simulink model "requriment_33"  (R2021a)
settings: Solver=FixedStepDiscrete  StartTime=0.0  StopTime=50  FixedStep=1  RelTol=1e-3
libraries: simulink x12
settings Model: DataDictionary=requriment_33.sldd  Creator=Rahul  LastModifiedBy=Rahul
settings ConfigComp: CovMetricSettings=dcmwe

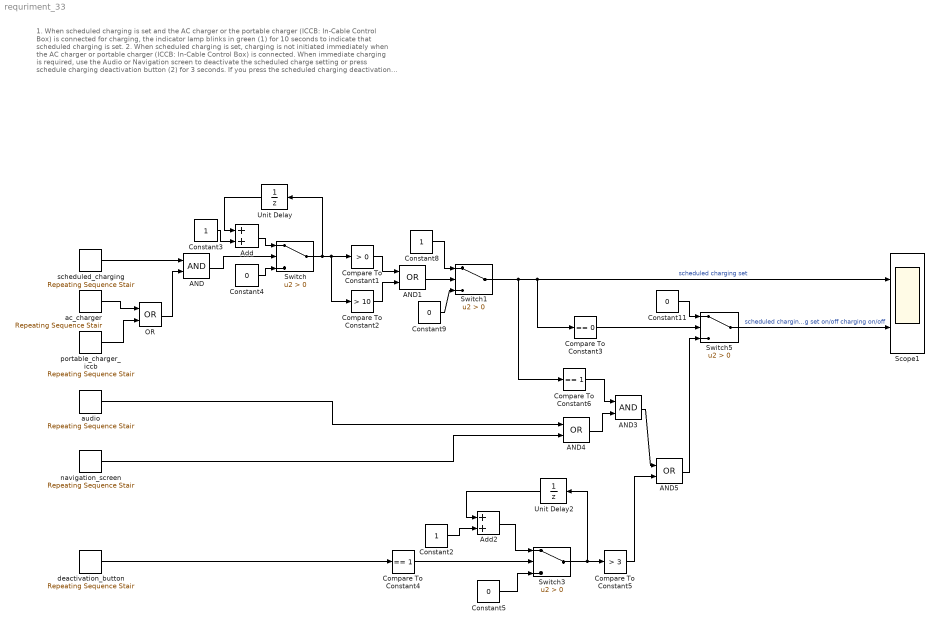
== system requriment_33 ==
  note: 1. When scheduled charging is set and the AC charger or the portable charger (ICCB: In-Cable Control Box) is connected for charging, the indicator lamp blinks in green (1) for 10 seconds to indicate
      | that scheduled charging is set.
      | 2. When scheduled charging is set, charging is not initiated immediately when the AC charger or portable charger (ICCB: In-Cable Control Box) is connected. When immediate charging is required,
      | use the Audio or Navigation screen to deactivate the scheduled charge setting
      | or press schedule charging deactivation button (2) for 3 seconds.
      | If you press the scheduled charging deactivation button (2) to immediately charge the battery,
      | charging must be initiated 3 minutes after the charging cable has been connected. When you press the scheduled charging deactivation button (2) for immediate charging, the schedul ed
      | charge setting
  AND : Logic  AllPortsSameDT=off  OutDataTypeStr=boolean
  AND1 : Logic  Operator=OR  AllPortsSameDT=off  OutDataTypeStr=boolean
  AND3 : Logic  AllPortsSameDT=off  OutDataTypeStr=boolean
  AND4 : Logic  Operator=OR  AllPortsSameDT=off  OutDataTypeStr=boolean
  AND5 : Logic  Operator=OR  AllPortsSameDT=off  OutDataTypeStr=boolean
  Add : Sum
  Add2 : Sum
  Compare To Constant1 : simulink/Logic and Bit Operations/Compare To Constant  relop=>  const=0  OutDataTypeStr=boolean
  Compare To Constant2 : simulink/Logic and Bit Operations/Compare To Constant  relop=>  const=10  OutDataTypeStr=boolean
  Compare To Constant3 : simulink/Logic and Bit Operations/Compare To Constant  relop===  const=0  OutDataTypeStr=boolean
  Compare To Constant4 : simulink/Logic and Bit Operations/Compare To Constant  relop===  const=1  OutDataTypeStr=boolean
  Compare To Constant5 : simulink/Logic and Bit Operations/Compare To Constant  relop=>  const=3  OutDataTypeStr=boolean
  Compare To Constant6 : simulink/Logic and Bit Operations/Compare To Constant  relop===  const=1  OutDataTypeStr=boolean
  Constant{4..5,9,11} (4 alike) : Constant  Value=0
  Constant2 : Constant
  Constant3 : Constant
  Constant8 : Constant
  OR : Logic  Operator=OR  AllPortsSameDT=off  OutDataTypeStr=boolean
  Scope1 : Scope  NumInputPorts=2
  Switch{,1,3,5} (4 alike) : Switch  Criteria=u2 > Threshold
  Unit Delay : UnitDelay  SampleTime=-1  HasFrameUpgradeWarning=on
  Unit Delay2 : UnitDelay  SampleTime=-1  HasFrameUpgradeWarning=on
  ac_charger : simulink/Sources/Repeating Sequence Stair  OutValues=[1 1 1 1 1 1 1 1 1 1 1 0 1 1 0 0 10 1 0 1 0 0 0 0]  tsamp=-1  OutMin=[]  OutMax=[]  OutDataTypeStr=double  OutputDataTypeScalingMode=double  OutDataType=fixdt(0,8)  ConRadixGroup=Best Precision: Vector-wise  OutScaling=2^-12
  audio : simulink/Sources/Repeating Sequence Stair  OutValues="[1 1 1 1 1 1 1 1 1 1 1 1 1 1 0 0 0  0 0 0  0 0 0 0]"  tsamp=-1  OutMin=[]  OutMax=[]  OutDataTypeStr=double  OutputDataTypeScalingMode=double  OutDataType=fixdt(0,8)  ConRadixGroup=Best Precision: Vector-wise  OutScaling=2^-12
  deactivation_button : simulink/Sources/Repeating Sequence Stair  OutValues="[1 1 1 1 1 1 1 1 1 1 1 1 1 1 0 0 0  0 0 0  0 0 0 0]"  tsamp=-1  OutMin=[]  OutMax=[]  OutDataTypeStr=double  OutputDataTypeScalingMode=double  OutDataType=fixdt(0,8)  ConRadixGroup=Best Precision: Vector-wise  OutScaling=2^-12
  navigation_screen : simulink/Sources/Repeating Sequence Stair  OutValues="[1 1 1 1 1 1 1 1 1 1 1 1 1 1 0 0 0  0 0 0  0 0 0 0]"  tsamp=-1  OutMin=[]  OutMax=[]  OutDataTypeStr=double  OutputDataTypeScalingMode=double  OutDataType=fixdt(0,8)  ConRadixGroup=Best Precision: Vector-wise  OutScaling=2^-12
  portable_charger_iccb : simulink/Sources/Repeating Sequence Stair  OutValues=[1 1 1 1 1 1 1 1 1 1 1 0 1 1 0 0 10 1 0 1 0 0 0 0]  tsamp=-1  OutMin=[]  OutMax=[]  OutDataTypeStr=double  OutputDataTypeScalingMode=double  OutDataType=fixdt(0,8)  ConRadixGroup=Best Precision: Vector-wise  OutScaling=2^-12
  scheduled_charging : simulink/Sources/Repeating Sequence Stair  OutValues=[1 1 1 1 1 1 1 1 1 1 1 1 1 1 0 0 10 1 0 1 0 0 0 0]  tsamp=-1  OutMin=[]  OutMax=[]  OutDataTypeStr=double  OutputDataTypeScalingMode=double  OutDataType=fixdt(0,8)  ConRadixGroup=Best Precision: Vector-wise  OutScaling=2^-12
  wires:
  Constant4/1 -> Switch/3
  ac_charger/1 -> OR/1
  portable_charger_iccb/1 -> OR/2
  AND/1 -> Switch/2
  scheduled_charging/1 -> AND/1
  Add/1 -> Switch/1
  OR/1 -> AND/2
  Constant3/1 -> Add/2
  Unit Delay/1 -> Add/1
  AND1/1 -> Switch1/2
  Constant9/1 -> Switch1/3
  Constant8/1 -> Switch1/1
  Compare To Constant1/1 -> AND1/1
  Compare To Constant2/1 -> AND1/2
  Switch/1 -> Compare To Constant2/1, Compare To Constant1/1, Unit Delay/1
  Unit Delay2/1 -> Add2/1
  Add2/1 -> Switch3/1
  Constant2/1 -> Add2/2
  Compare To Constant4/1 -> Switch3/2
  Switch3/1 -> Unit Delay2/1, Compare To Constant5/1
  Constant5/1 -> Switch3/3
  Compare To Constant6/1 -> AND3/1
  audio/1 -> AND4/1
  navigation_screen/1 -> AND4/2
  AND4/1 -> AND3/2
  Compare To Constant3/1 -> Switch5/2
  Constant11/1 -> Switch5/1
  Switch5/1 -> Scope1/2  "scheduled charging set on/off charging on/off"
  deactivation_button/1 -> Compare To Constant4/1
  AND3/1 -> AND5/1
  Compare To Constant5/1 -> AND5/2
  AND5/1 -> Switch5/3
  Switch1/1 -> Compare To Constant3/1, Scope1/1, Compare To Constant6/1  "scheduled charging set"
